simulink model "lab11"  (Simulink 8.5)
settings: Solver=ode45  StartTime=0.0  StopTime=10000000  RelTol=1e-3
settings Model: Creator=Meteo  LastModifiedBy=Meteo
settings DataIOCC: SignalLoggingSaveFormat=Dataset
settings OptimizationCC: ExpressionDepthLimit=128
settings DebuggingCC: UnderspecifiedInitializationDetection=Simplified  MergeDetectMultiDrivingBlocksExec=error  FcnCallInpInsideContextMsg=EnableAllAsError  StateNameClashWarn=none
settings GRTTargetCC: CombineOutputUpdateFcns=on  GRTInterface=off

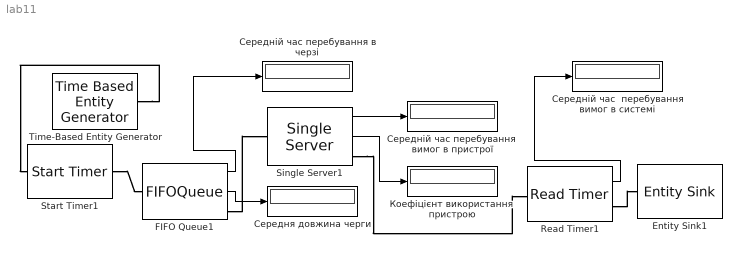
== system lab11 ==
  Entity Sink1 : EntitySink
  FIFO Queue1 : FIFOQueue  StatAverageWait=on  StatAverageQueueLength=on
      settings: OutputPortMap=o2,o3
  Read Timer1 : ReadTimer  StatAverageTimeElapsed=on
      settings: OutputPortMap=o3
  Single Server1 : SingleServer  RequirementInfo="{}  %GIDa_6e44fa00_f48c_42b0_8a76_4938543c7af8"  ServiceTime=17  StatAverageWait=on  StatUtilization=on
      settings: OutputPortMap=o4,o5
  Start Timer1 : StartTimer
  Time-Based Entity Generator : TimeBasedEntityGenerator  Distribution=Exponential  Period=27  InitialSeed=64574  Mean=27
  Коефіцієнт використання  пристрою : Display
  Середня довжина черги : Display
  Середній час  перебування вимог в системі : Display
  "Середній час перебування  вимог в пристрої " : Display
  Середній час перебування в черзі : Display
  wires:
  Single Server1/1 -> "Середній час перебування  вимог в пристрої "/1
  Read Timer1/1 -> Середній час  перебування вимог в системі/1
  Single Server1/2 -> Коефіцієнт використання  пристрою/1
  FIFO Queue1/2 -> Середня довжина черги/1
  FIFO Queue1/1 -> Середній час перебування в черзі/1
  connections:
  Single Server1/RConn1 -- Read Timer1/LConn1
  FIFO Queue1/RConn1 -- Single Server1/LConn1
  Start Timer1/RConn1 -- FIFO Queue1/LConn1
  Read Timer1/RConn1 -- Entity Sink1/LConn1
  Time-Based Entity Generator/RConn1 -- Start Timer1/LConn1
